simulink model "Trajectory"  (R2025a)
settings: Solver=ode4  StartTime=0.0  StopTime=60  FixedStep=0.01  RelTol=1e-3

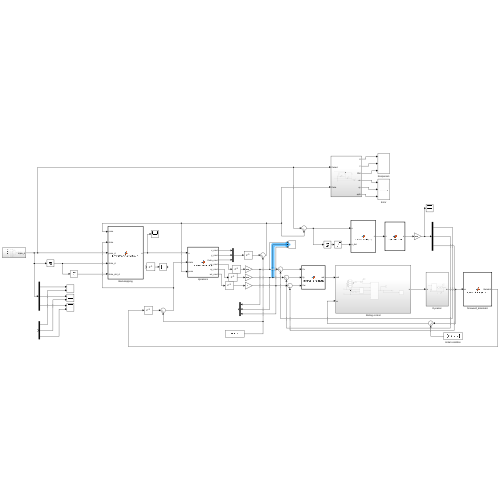
[thumbnail: Simulink's stored preview of the top-level diagram]
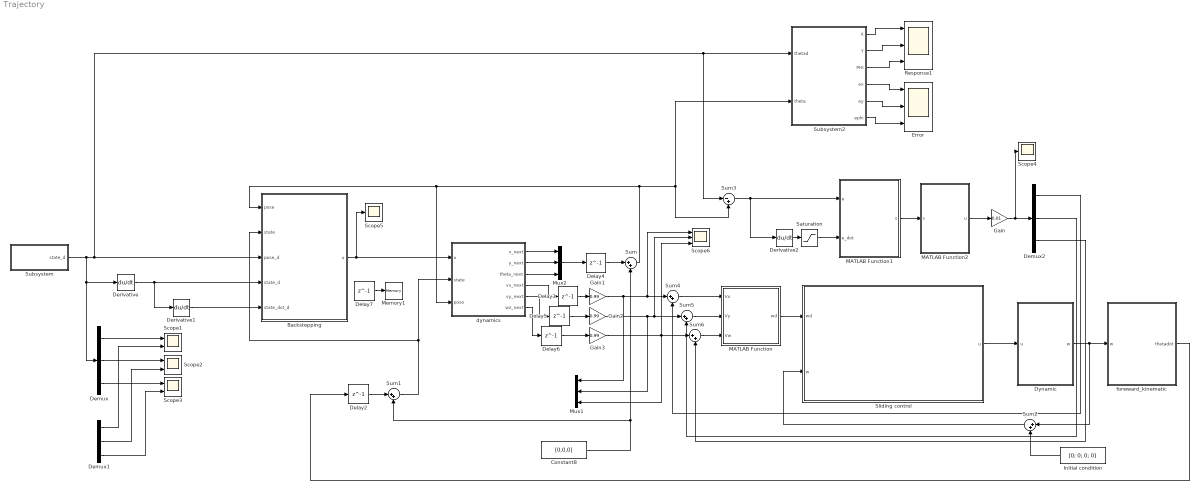
== system Trajectory ==
  Backstepping : MATLAB Function  TreatAsAtomicUnit=on
  Constant8 : Constant  Value=[0,0,0]  VectorParams1D=off
  Delay{2..7} (6 alike) : Delay  DelayLength=1  InitialCondition=0
  Demux : Demux  Outputs=3
  Demux1 : Demux  Outputs=3
  Demux2 : Demux  Outputs=3
  Derivative : Derivative
  Derivative1 : Derivative
  Derivative2 : Derivative
  Dynamic : Subsystem
  "Error " : Scope  NumInputPorts=3
      settings: ActiveDisplayYMinimum=-0.69401065549567176  ActiveDisplayYMaximum=2.299334517277297
  Gain : Gain  Gain=0.01
  Gain1 : Gain  Gain=0.99
  Gain2 : Gain  Gain=0.99
  Gain3 : Gain  Gain=0.99
  Initial condition : Constant  Value=[0; 0; 0; 0]
  MATLAB Function : MATLAB Function  TreatAsAtomicUnit=on
  MATLAB Function1 : MATLAB Function  TreatAsAtomicUnit=on
  MATLAB Function2 : MATLAB Function  TreatAsAtomicUnit=on
  Memory1 : Memory
  Mux1 : Mux  Inputs=3
  Mux2 : Mux  Inputs=3
  Response1 : Scope  NumInputPorts=3
      settings: ActiveDisplayYMinimum=-2.5374628262899326  ActiveDisplayYMaximum=2.7721218113487729  DataLoggingVariableName=ScopeData7
  Saturation : Saturate  UpperLimit=500  LowerLimit=-500
  Scope1 : Scope  NumInputPorts=2
      settings: ActiveDisplayYMinimum=-1  ActiveDisplayYMaximum=1
  Scope2 : Scope  NumInputPorts=2
      settings: ActiveDisplayYMinimum=-1  ActiveDisplayYMaximum=1  DataLoggingVariableName=ScopeData2
  Scope3 : Scope  NumInputPorts=2
      settings: ActiveDisplayYMinimum=-1  ActiveDisplayYMaximum=1  DataLoggingVariableName=ScopeData3
  Scope4 : Scope
      settings: ActiveDisplayYMinimum=-151.71373469733481  ActiveDisplayYMaximum=484.35954203685446  DataLoggingVariableName=ScopeData8
  Scope5 : Scope
      settings: ActiveDisplayYMinimum=-151.71373469733481  ActiveDisplayYMaximum=484.35954203685446  DataLoggingVariableName=ScopeData5
  Scope6 : Scope  NumInputPorts=3
      settings: ActiveDisplayYMinimum=-151.71373469733481  ActiveDisplayYMaximum=484.35954203685446  DataLoggingVariableName=ScopeData9
  Sliding control : Subsystem
  Subsystem : Subsystem
  Subsystem2 : Subsystem
  Sum{,1..2,4..6} (6 alike) : Sum  Inputs=|++
  Sum3 : Sum  Inputs=|-+
  dynamics : MATLAB Function  TreatAsAtomicUnit=on
  forwward_kinematic : MATLAB Function  TreatAsAtomicUnit=on
  wires:
  Backstepping/1(u) -> dynamics/1(u), Scope5/1
  dynamics/1(x_next) -> Mux2/1
  dynamics/2(y_next) -> Mux2/2
  dynamics/3(theta_next) -> Mux2/3
  Constant8/1 -> Sum/2, Sum1/2
  Mux2/1 -> Delay4/1
  Delay2/1 -> Sum1/1
  Subsystem/1(state_d) -> Subsystem2/1(thetad), Sum3/1, Backstepping/3(pose_d), Derivative/1, Demux/1
  Derivative/1 -> Derivative1/1, Backstepping/4(state_d)
  Derivative1/1 -> Backstepping/5(state_dot_d)
  Demux/1 -> Scope1/1
  Demux/2 -> Scope2/1
  Demux/3 -> Scope3/1
  Demux1/1 -> Scope1/2
  Demux1/2 -> Scope2/2
  Demux1/3 -> Scope3/2
  Sliding control/1(u) -> Dynamic/1(u)
  Dynamic/1(w) -> Sum2/1, forwward_kinematic/1(w)
  MATLAB Function/1(wd) -> Sliding control/1(wd)
  Initial condition/1 -> Sum2/2
  Subsystem2/3(PHI) -> Response1/3
  Subsystem2/2(Y) -> Response1/2
  Subsystem2/1(X) -> Response1/1
  Subsystem2/4(ex) -> "Error "/1
  Subsystem2/5(ey) -> "Error "/2
  Subsystem2/6(ephi) -> "Error "/3
  forwward_kinematic/1(thetadot) -> Delay2/1
  Sum2/1 -> Sliding control/2(w)
  dynamics/4(vx_next) -> Delay3/1
  dynamics/5(vy_next) -> Delay5/1
  dynamics/6(wz_next) -> Delay6/1
  Delay3/1 -> Gain1/1
  Delay5/1 -> Gain2/1
  Delay6/1 -> Gain3/1
  Delay4/1 -> Sum/1
  Sum/1 -> dynamics/3(pose), Backstepping/1(pose), Sum3/2, Subsystem2/2(theta)
  Sum1/1 -> dynamics/2(state), Backstepping/2(state)
  MATLAB Function1/1(s) -> MATLAB Function2/1(s)
  Derivative2/1 -> Saturation/1
  Saturation/1 -> MATLAB Function1/2(e_dot)
  Sum3/1 -> MATLAB Function1/1(e), Derivative2/1
  MATLAB Function2/1(u) -> Gain/1
  Sum6/1 -> MATLAB Function/3(Vw)
  Sum5/1 -> MATLAB Function/2(Vy)
  Sum4/1 -> MATLAB Function/1(Vx)
  Demux2/1 -> Sum4/2
  Demux2/2 -> Sum5/2
  Demux2/3 -> Sum6/2
  Gain/1 -> Scope4/1, Demux2/1
  Gain1/1 -> Scope6/1, Sum4/1, Mux1/1
  Gain2/1 -> Sum5/1, Scope6/2, Mux1/2
  Gain3/1 -> Scope6/3, Sum6/1, Mux1/3
  Delay7/1 -> Memory1/1

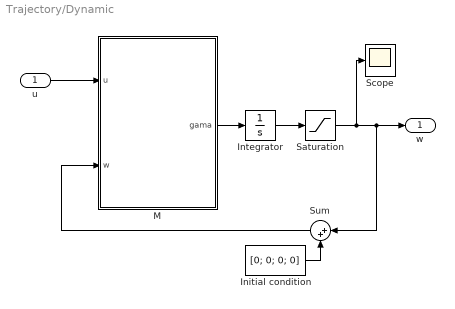
== system Trajectory/Dynamic ==
  u : Inport
  Initial condition : Constant  Value=[0; 0; 0; 0]
  Integrator : Integrator
  M : MATLAB Function  TreatAsAtomicUnit=on
  Saturation : Saturate  UpperLimit=300  LowerLimit=-300
  Scope : Scope
      settings: ActiveDisplayYMinimum=-59.566364364043068  ActiveDisplayYMaximum=58.139141196553538  DataLoggingVariableName=ScopeData6
  Sum : Sum  Inputs=|++
  w : Outport
  wires:
  u/1 -> M/1(u)
  Integrator/1 -> Saturation/1
  Saturation/1 -> Scope/1, Sum/1, w/1
  Sum/1 -> M/2(w)
  Initial condition/1 -> Sum/2
  M/1(gama) -> Integrator/1

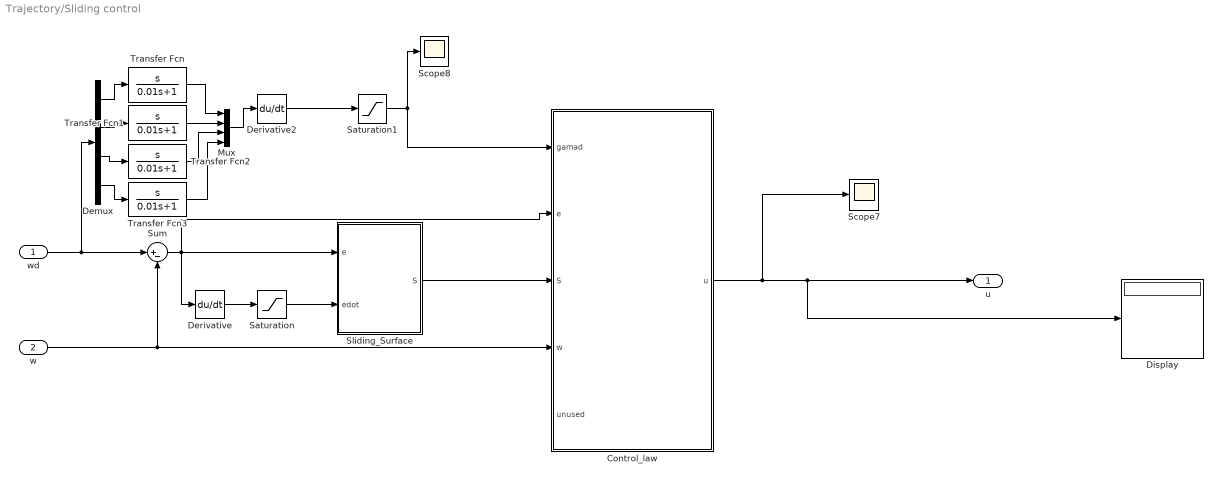
== system Trajectory/Sliding control ==
  wd : Inport
  w : Inport  Port=2
  Control_law : MATLAB Function  TreatAsAtomicUnit=on
  Demux : Demux
  Derivative : Derivative
  Derivative2 : Derivative
  Display : Display
  Mux : Mux
  Saturation : Saturate  UpperLimit=500  LowerLimit=-500
  Saturation1 : Saturate  UpperLimit=500  LowerLimit=-500
  Scope7 : Scope
      settings: ActiveDisplayYMinimum=-5242.26134  ActiveDisplayYMaximum=21074.01148  DataLoggingVariableName=ScopeData3
  Scope8 : Scope
      settings: ActiveDisplayYMinimum=-625  ActiveDisplayYMaximum=625  DataLoggingVariableName=ScopeData4
  Sliding_Surface : MATLAB Function  TreatAsAtomicUnit=on
  Sum : Sum  Inputs=|+-
  Transfer Fcn{,1..3} (4 alike) : TransferFcn  Numerator=[1 0]  Denominator=[0.01 1]
  u : Outport
  wires:
  w/1 -> Control_law/4(w), Sum/2
  Sum/1 -> Derivative/1, Control_law/2(e), Sliding_Surface/1(e)
  Derivative/1 -> Saturation/1
  wd/1 -> Demux/1, Sum/1
  Saturation/1 -> Sliding_Surface/2(edot)
  Saturation1/1 -> Scope8/1, Control_law/1(gamad)
  Derivative2/1 -> Saturation1/1
  Sliding_Surface/1(S) -> Control_law/3(S)
  Control_law/1(u) -> Scope7/1, Display/1, u/1
  Demux/1 -> Transfer Fcn/1
  Demux/4 -> Transfer Fcn3/1
  Demux/3 -> Transfer Fcn2/1
  Demux/2 -> Transfer Fcn1/1
  Transfer Fcn/1 -> Mux/1
  Transfer Fcn1/1 -> Mux/2
  Transfer Fcn2/1 -> Mux/3
  Transfer Fcn3/1 -> Mux/4
  Mux/1 -> Derivative2/1

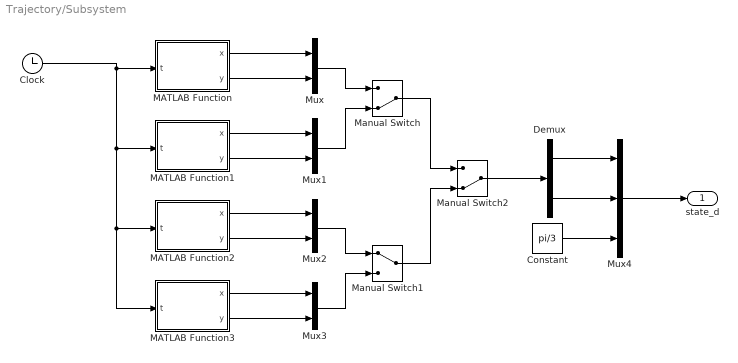
== system Trajectory/Subsystem ==
  Clock : Clock
  Constant : Constant  Value=pi/3
  Demux : Demux  Outputs=2
  MATLAB Function : MATLAB Function  TreatAsAtomicUnit=on
  MATLAB Function1 : MATLAB Function  TreatAsAtomicUnit=on
  MATLAB Function2 : MATLAB Function  TreatAsAtomicUnit=on
  MATLAB Function3 : MATLAB Function  TreatAsAtomicUnit=on
  Manual Switch : ManualSwitch  CurrentSetting=0
  Manual Switch1 : ManualSwitch
  Manual Switch2 : ManualSwitch  CurrentSetting=0
  Mux{,1..3} (4 alike) : Mux  Inputs=2
  Mux4 : Mux  Inputs=3
  state_d : Outport
  wires:
  Clock/1 -> MATLAB Function3/1(t), MATLAB Function2/1(t), MATLAB Function1/1(t), MATLAB Function/1(t)
  Mux2/1 -> Manual Switch1/1
  Mux3/1 -> Manual Switch1/2
  Manual Switch1/1 -> Manual Switch2/2
  Manual Switch/1 -> Manual Switch2/1
  Mux/1 -> Manual Switch/1
  Mux1/1 -> Manual Switch/2
  Manual Switch2/1 -> Demux/1
  Demux/2 -> Mux4/2
  Demux/1 -> Mux4/1
  MATLAB Function3/1(x) -> Mux3/1
  MATLAB Function3/2(y) -> Mux3/2
  MATLAB Function2/1(x) -> Mux2/1
  MATLAB Function2/2(y) -> Mux2/2
  MATLAB Function1/1(x) -> Mux1/1
  MATLAB Function1/2(y) -> Mux1/2
  MATLAB Function/1(x) -> Mux/1
  MATLAB Function/2(y) -> Mux/2
  Constant/1 -> Mux4/3
  Mux4/1 -> state_d/1

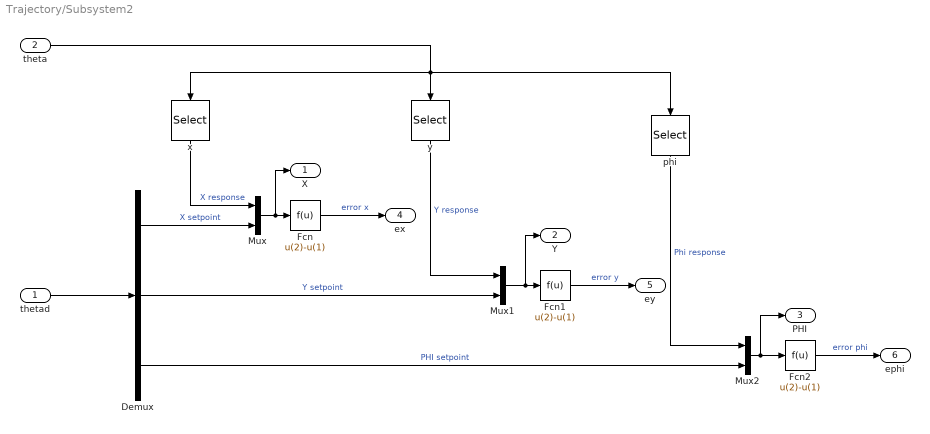
== system Trajectory/Subsystem2 ==
  thetad : Inport
  theta : Inport  Port=2
  Demux : Demux  Outputs=3
  Fcn : Fcn  Expr=u(2)-u(1)
  Fcn1 : Fcn  Expr=u(2)-u(1)
  Fcn2 : Fcn  Expr=u(2)-u(1)
  Mux : Mux  Inputs=2
  Mux1 : Mux  Inputs=2
  Mux2 : Mux  Inputs=2
  phi : Selector  InputPortWidth=3  IndexOptions=Index vector (dialog)  Indices=[3]  OutputSizes=1
  x : Selector  InputPortWidth=3  IndexOptions=Index vector (dialog)  Indices=[1]  OutputSizes=1
  y : Selector  InputPortWidth=3  IndexOptions=Index vector (dialog)  Indices=[2]  OutputSizes=1
  X : Outport
  Y : Outport  Port=2
  PHI : Outport  Port=3
  ex : Outport  Port=4
  ey : Outport  Port=5
  ephi : Outport  Port=6
  wires:
  thetad/1 -> Demux/1
  theta/1 -> x/1, phi/1, y/1
  Demux/1 -> Mux/2  "X setpoint"
  x/1 -> Mux/1  "X response"
  y/1 -> Mux1/1  "Y response"
  Demux/2 -> Mux1/2  "Y setpoint"
  Demux/3 -> Mux2/2  "PHI setpoint"
  phi/1 -> Mux2/1  "Phi response"
  Mux/1 -> Fcn/1, X/1
  Mux1/1 -> Fcn1/1, Y/1
  Fcn/1 -> ex/1  "error x"
  Fcn1/1 -> ey/1  "error y"
  Fcn2/1 -> ephi/1  "error phi"
  Mux2/1 -> Fcn2/1, PHI/1

== matlab function Trajectory/Sliding control/Sliding_Surface ==
  data: e input; S output; edot input
function S = Sliding_surface(e, edot)
%Khai báo giá trị
lamda1 = 6;
lamda2 = 6;
lamda3 = 6;
lamda4 = 6;
%Tính toán
delta = diag ([lamda1 lamda2 lamda3 lamda4]);
S = edot + delta*e;

== matlab function Trajectory/forwward_kinematic ==
  data: w input; thetadot output
function thetadot = forward_kinematic(w)
%Khai báo giá trị
R = 0.035;
L = 0.1; W = 0.1;

%Tính toán
Jod = [-1 1 -1 1;
        1 1 1 1;
      1/(L+W) -1/(L+W) -1/(L+W) 1/(L+W)];
thetadot = (R/4)*Jod*w;

== matlab function Trajectory/Dynamic/M ==
  data: u input; gama output; w input
function gama = Dynamic(u, w)
%Khai báo giá trị
m = 6; R = 0.035;
L = 0.1; W = 0.1;
Iz = 0.22; Iw = 0.02328;
Dw_value = 0.4;
Dw = diag([Dw_value Dw_value Dw_value Dw_value]);
f = 10;

%Tính A,B,C,D
A = m*(R^2)/8;
B = (Iz*(R^2))/(16*(W+L)^2);
C = A+B+Iw;
D = A-B;

%Tính M0
M0 = [C -B B D;
     -B C D B;
     B D C -B;
     D B -B C];

%Tính Q
% Q = u - (m*9.8/4)*f*sign(w);

% Gia tốc góc 4 bánh xe
Eq = [2; 2; 2; 2];
H0 = M0\Dw;

% gama = M0\(Q-Dw*w);
%E = [2 2 2 2; 2 2 2 2; 2 2 2 2; 2 2 2 2];
% gama = M0\u - M0\Eq - M0\Dw*w;
gama = M0\u - M0\Dw*w;

== matlab function Trajectory/MATLAB Function1 ==
  data: e input; s output; e_dot input
function s  = sliding_surface(e,e_dot)

denta = 0.4;

% sliding_surface
s = e_dot + denta*e;

== matlab function Trajectory/MATLAB Function2 ==
  data: s input; u output
function u = control_law(s)
% he so k
k0 = 4;
k1 = 4;

% tin hieu dieu khien U_s
u = k0*s + k1*tanh(s);

== matlab function Trajectory/dynamics ==
  data: u input; x_next output size=1; state input; pose input; y_next output size=1; theta_next output size=1; vx_next output size=1; vy_next output size=1; wz_next output size=1
function [x_next, y_next, theta_next, vx_next, vy_next, wz_next] = RobotDynamics(u, state, pose)
% u: [Fx; Fy; Mz] - lực điều khiển từ Backstepping
% state: [vx; vy; wz] - vận tốc hiện tại
% pose: [x; y; theta] - vị trí hiện tại
% Ts: thời gian lấy mẫu

% Thông số hệ thống
m = 6;
L1 = 0.1; L2 = 0.1;
Iz = 0.22 + 0.02328;
Ts = 0.01;
% Tách input
Fx = u(1);
Fy = u(2);
Mz = u(3);

vx = state(1);
vy = state(2);
wz = state(3);

x = pose(1);
y = pose(2);
theta = pose(3);

% Ma trận quán tính
D = [ m,      0,       -m*L1;
      0,      m,        m*L2;
     -m*L1,  m*L2,    Iz + m*(L1^2 + L2^2)];

% Vector vận tốc
zeta = [vx; vy; wz];

% Nhiễu
n_zeta = [
    -m * (vy + L2 * wz);
     m * (vx - L1 * wz);
     m * wz * (L2 * vx + L1 * vy)
];

% Gia tốc
zeta_dot = D \ (u - n_zeta); % zeta_dot = [ax; ay; wz_dot]

% Tích phân Euler
vx_next = vx + Ts * zeta_dot(1);
vy_next = vy + Ts * zeta_dot(2);
wz_next = wz + Ts * zeta_dot(3);

% Kinematic: dx/dt = cos*vx - sin*vy (chuyển từ body -> global)
x_dot = cos(theta)*vx - sin(theta)*vy;
y_dot = sin(theta)*vx + cos(theta)*vy;
theta_dot = wz;

x_next = x + Ts * x_dot;
y_next = y + Ts * y_dot;
theta_next = wrapToPi(theta + Ts * theta_dot);

end

== matlab function Trajectory/MATLAB Function ==
  data: Vx input; wd output; Vy input; Vw input
function wd = inverse_kinematic(Vx,Vy,Vw)
%Khai báo giá trị
R = 0.035;
L = 0.1; W = 0.1;

%Tính toán
theta = [Vx; Vy; Vw];
J = [-1 1 L+W;
      1 1 -(L+W);
     -1 1 -(L+W);
      1 1 L+W];
wd = (1/R)*J*theta;

== matlab function Trajectory/Subsystem/MATLAB Function ==
  data: x output; t input; y output
function [x,y] = rectangle(t)
a = 2;
b = 1;
T = mod(t,20);

if T < 2.5
    x = (a/2)*(T/2.5);
    y = b/2;
elseif T >= 2.5 && T < 7.5
    x = a/2;
    y = (b/2)-b*(T-2.5)/5; 
elseif T >= 7.5 && T < 12.5
    x = (a/2)-a*(T-7.5)/5;
    y = -b/2;
elseif T >= 12.5 && T < 17.5
    x = -a/2;
    y = -(b/2)+b*(T-12.5)/5;
elseif T >= 17.5 && T < 20
    x = -a/2+(a/2)*(T-17.5)/2.5;
    y = b/2;
else 
    x = 0;
    y = b/2;
end

== matlab function Trajectory/Backstepping ==
  data: pose input; u output; state input; pose_d input; state_d input; state_dot_d input
function u = BacksteppingController(pose,state,pose_d,state_d,state_dot_d)

% Assign value
x            = pose(1);
y            = pose(2);
theta        = pose(3);

x_dot        = state(1);
y_dot        = state(2);
theta_dot    = state(3);

x_d          = pose_d(1);
y_d          = pose_d(2);
theta_d      = pose_d(3);

x_dot_d      = state_d(1);
y_dot_d      = state_d(2);
theta_dot_d  = state_d(3);

x_ddot_d     = state_dot_d(1);
y_ddot_d     = state_dot_d(2);
theta_ddot_d = state_dot_d(3);
% Tham số hệ thống
k1 = 6;
k2 = 6;
m = 6;
L1 = 0.1; L2 = 0.1;
I_z = 0.22 + 0.02328;

% Sai số vị trí
e1 = [x_d - x;
      y_d - y;
      wrapToPi(theta_d - theta)];

% Sai số vận tốc
e2 = zeros(3,1); % Tạm thời khởi tạo

% Ma trận Jacobian
J = [cos(theta), -sin(theta), 0;
     sin(theta),  cos(theta), 0;
          0,          0,      1];

J_inv = pinv(J);

% Vận tốc tham chiếu
zeta_d = J_inv * ( [x_dot_d; y_dot_d; theta_dot_d] + k1 * e1 );

% Tính đạo hàm sai số vị trí
%e1_dot = [x_dot_d - (cos(theta)*x_dot + -sin(theta)*y_dot);
 %         y_dot_d - (sin(theta)*x_dot + cos(theta)*y_dot);
   %       theta_dot_d - theta_dot];
e1_dot = [x_dot_d - x_dot;
          y_dot_d - y_dot;
          theta_dot_d - theta_dot];
% Đạo hàm vận tốc tham chiếu
zeta_dot_d = J_inv * ( [x_ddot_d; y_ddot_d; theta_ddot_d] + k1 * e1_dot );

% Sai số vận tốc
e2 = zeta_d - [x_dot; y_dot; theta_dot];

% Ma trận quán tính
D = [ m,      0,       -m*L1;
      0,      m,        m*L2;
     -m*L1,  m*L2,    I_z + m*(L1^2 + L2^2)];

% Nhiễu
n_zeta = [
    -m * (y_dot + L2 * theta_dot);
     m * (x_dot - L1 * theta_dot);
     m * theta_dot * (L2 * x_dot + L1 * y_dot)
];

% Điều khiển
u = D * (k2 * e2 + zeta_dot_d + J' * e1) + n_zeta;

end

== matlab function Trajectory/Subsystem/MATLAB Function1 ==
  data: x output; t input; y output
function [x,y] = circle(t)
Radius = 1;
T = 20;
x = Radius*cos(2*pi*t/T);
y = Radius*sin(2*pi*t/T);

== matlab function Trajectory/Subsystem/MATLAB Function2 ==
  data: x output; t input; y output
function [x,y] = ellipse(t)
a = 2;
b = 1;
T = 20;
x = a*cos(2*pi*t/T);
y = b*sin(2*pi*t/T);

== matlab function Trajectory/Subsystem/MATLAB Function3 ==
  data: x output; t input; y output
function [x,y] = path8(t)
a = 2;
b = 2;
x = a*sin(2*pi/10*t) + 0; % X-axis desired value (pixel)
y = b*cos(2*pi/20*t) + 0; % Y-axis desired value (pixel)

== matlab function Trajectory/Sliding control/Control_law ==
  data: gamad input; e input; u output; S input; w input; unused input
function u = control_law(gamad, e, S, w, ~)
% control_law - Sliding mode control law matching eq. (17)
% gamad:   qddot_d (4x1)
% e:       e_M = qdot_d - qdot (4x1)
% S:       sliding surface (4x1)
% w:       qdot (4x1)
% last arg unused placeholder

% params
m = 6; R = 0.035;
L = 0.1; W = 0.1;
Iz = 0.22; Iw = 0.02328;
Dw_val = 0.4;
Dw = diag([Dw_val Dw_val Dw_val Dw_val]);

lamda1 = 6;
lamda2 = 6;
lamda3 = 6;
lamda4 = 6;

lamda11 = 9;
lamda12 = 9;
lamda13 = 9;
lamda14 = 9;

lamda21 = 9;
lamda22 = 9;
lamda23 = 9;
lamda24 = 9;

%Tính A,B,C,D
A = m*(R^2)/8;
B = (Iz*(R^2))/(16*(W+L)^2);
C = A+B+Iw;
D = A-B;

%Tính M0
M0 = [C -B B D;
     -B C D B;
     B D C -B;
     D B -B C];

%Tính ma trận các tham số điều khiển
delta = diag ([lamda1 lamda2 lamda3 lamda4]);
lamda1s = diag ([lamda11 lamda12 lamda13 lamda14]);
lamda2s = diag ([lamda21 lamda22 lamda23 lamda24]);

%Tính H0
H0 = M0\Dw;

%Tính tín hiệu điều khiển u
     u = M0*(lamda1s*S+lamda2s*tanh(S)+delta*e+gamad+H0*w);
% Eq = [2; 2; 2; 2];
%  fz = delta*e+gamad+H0*w + M0\Eq - f;
%    u = M0*(lamda1s*S+lamda2s*sign(S)+f); %ueq + urbf

end
